simulink model "Controlador_Virtual_velocidade"  (R2021a)
settings: Solver=VariableStepAuto  StartTime=0.0  StopTime=10  RelTol=1e-3
undefined symbols (not defined in the file or in its folder): D1, D2, D3, id, iq, Kt, w
settings Model: Creator=migue  LastModifiedBy=migue

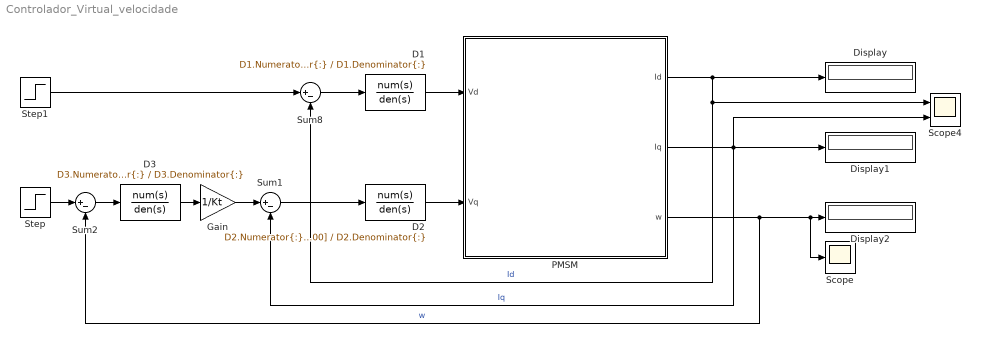
== system Controlador_Virtual_velocidade ==
  D1 : TransferFcn  Numerator=D1.Numerator{:}  Denominator=D1.Denominator{:}
  D2 : TransferFcn  Numerator=D2.Numerator{:}.*[1 1000]  Denominator=D2.Denominator{:}
  D3 : TransferFcn  Numerator=D3.Numerator{:}  Denominator=D3.Denominator{:}
  Display : Display
  Display1 : Display
  Display2 : Display
  Gain : Gain  Gain=1/Kt
  PMSM : Subsystem  mask{R=0.16, L=1.3e-4, N=10, J=1.8e-4, b=1e-5, lamb=0.06, Kt=0.095}
      mask prompts: R "Resitência (R)"; L "Indutância(L)"; N "Nº de par de polos(N)"; J "coeficiente(J)"; b "coeficiente(b)"; lamb "(lamb)"; Kt "(Kt)"
  Scope : Scope
  Scope4 : Scope  NumInputPorts=2
  Step : Step  After=100  SampleTime=0
  Step1 : Step  After=0  SampleTime=0
  Sum1 : Sum  Inputs=|+-
  Sum2 : Sum  Inputs=|+-
  Sum8 : Sum  Inputs=|+-
  wires:
  PMSM/1(Id) -> Scope4/1, Sum8/2, Display/1  "Id"
  D2/1 -> PMSM/2(Vq)
  Sum1/1 -> D2/1
  D1/1 -> PMSM/1(Vd)
  Sum8/1 -> D1/1
  PMSM/2(Iq) -> Display1/1, Sum1/2, Scope4/2  "Iq"
  Sum2/1 -> D3/1
  PMSM/3(w) -> Scope/1, Display2/1, Sum2/2  "w"
  Step/1 -> Sum2/1
  D3/1 -> Gain/1
  Gain/1 -> Sum1/1
  Step1/1 -> Sum8/1

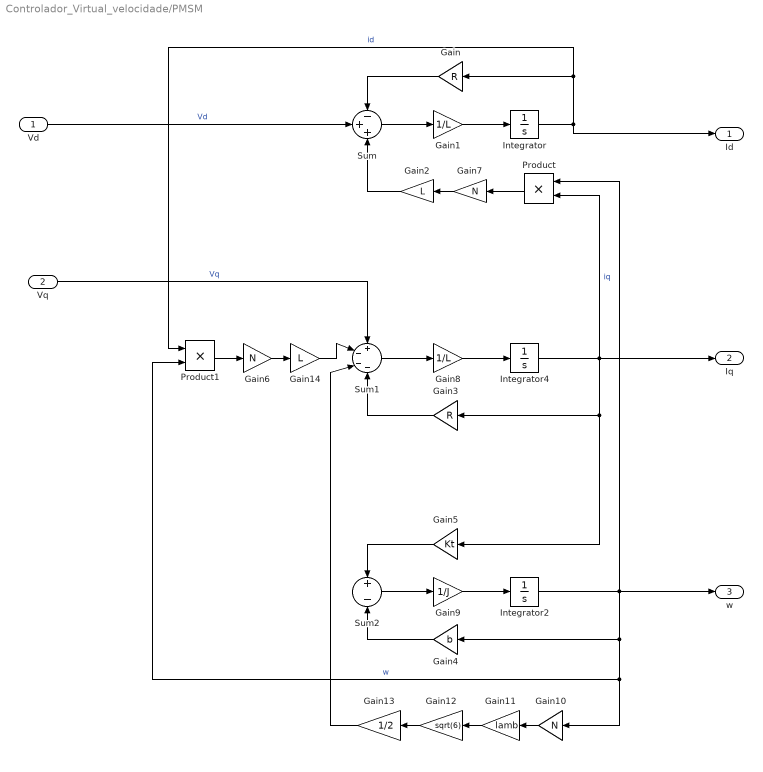
== system Controlador_Virtual_velocidade/PMSM ==
  Vd : Inport
  Vq : Inport  Port=2
  Gain : Gain  Gain=R
  Gain1 : Gain  Gain=1/L
  Gain10 : Gain  Gain=N
  Gain11 : Gain  Gain=lamb
  Gain12 : Gain  Gain=sqrt(6)
  Gain13 : Gain  Gain=1/2
  Gain14 : Gain  Gain=L
  Gain2 : Gain  Gain=L
  Gain3 : Gain  Gain=R
  Gain4 : Gain  Gain=b
  Gain5 : Gain  Gain=Kt
  Gain6 : Gain  Gain=N
  Gain7 : Gain  Gain=N
  Gain8 : Gain  Gain=1/L
  Gain9 : Gain  Gain=1/J
  Integrator : Integrator  InitialCondition=id
  Integrator2 : Integrator  InitialCondition=w
  Integrator4 : Integrator  InitialCondition=iq
  Product : Product
  Product1 : Product
  Sum : Sum  Inputs=-++
  Sum1 : Sum  Inputs=+---
  Sum2 : Sum  Inputs=+-
  Id : Outport
  Iq : Outport  Port=2
  w : Outport  Port=3
  wires:
  Integrator4/1 -> Iq/1, Product/2, Gain3/1, Gain5/1  "iq"
  Integrator/1 -> Gain/1, Product1/1, Id/1  "id"
  Gain8/1 -> Integrator4/1
  Sum1/1 -> Gain8/1
  Product1/1 -> Gain6/1
  Gain/1 -> Sum/1
  Sum2/1 -> Gain9/1
  Integrator2/1 -> w/1, Product/1, Gain10/1, Product1/2, Gain4/1  "w"
  Gain5/1 -> Sum2/1
  Vd/1 -> Sum/2  "Vd"
  Gain9/1 -> Integrator2/1
  Gain1/1 -> Integrator/1
  Sum/1 -> Gain1/1
  Gain4/1 -> Sum2/2
  Gain3/1 -> Sum1/4
  Gain11/1 -> Gain12/1
  Gain10/1 -> Gain11/1
  Product/1 -> Gain7/1
  Vq/1 -> Sum1/1  "Vq"
  Gain12/1 -> Gain13/1
  Gain13/1 -> Sum1/3
  Gain6/1 -> Gain14/1
  Gain7/1 -> Gain2/1
  Gain2/1 -> Sum/3
  Gain14/1 -> Sum1/2
